simulink library "speedgoatlib_mscp"  (R2024b)
settings: Solver=VariableStepAuto  StartTime=0.0  StopTime=10.0  RelTol=1e-3
libraries: slrealtimeethercatlib x517, simulink x316, hdlsllib x168, $bdroot x11, slrealtimeutilitieslib x1
(part 3 of 5)

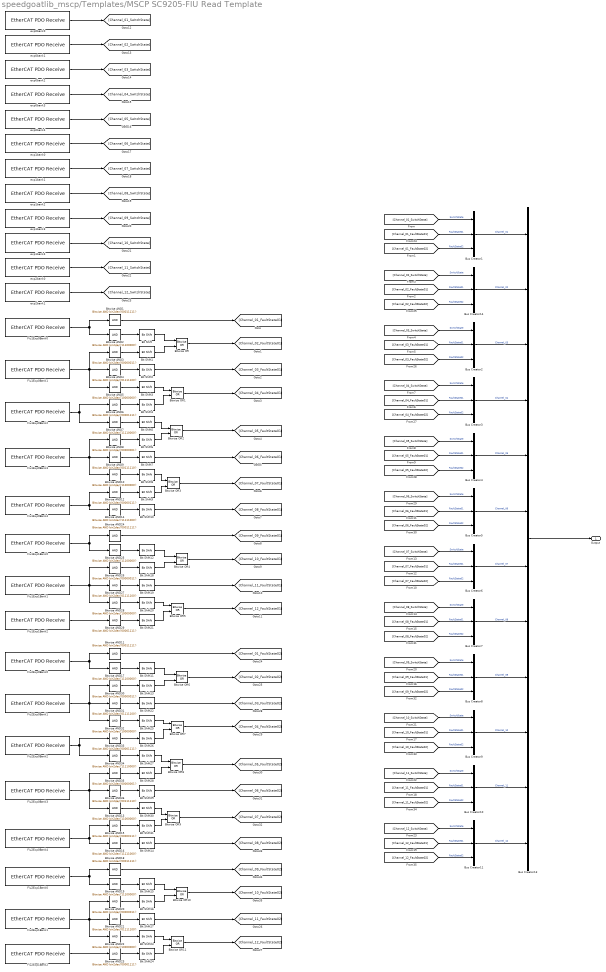
== system speedgoatlib_mscp/Templates/MSCP SC9205-FIU Read Template ==
  Bit Shift{,11..12,15} (4 alike) : hdlsllib/Logic and Bit Operations/Bit Shift  mode=Shift Right Logical  N=5
  Bit Shift{1,13,16,18} (4 alike) : hdlsllib/Logic and Bit Operations/Bit Shift  mode=Shift Left Logical  N=3
  Bit Shift10 : hdlsllib/Logic and Bit Operations/Bit Shift  mode=Shift Right Logical  N=3
  Bit Shift14 : hdlsllib/Logic and Bit Operations/Bit Shift  mode=Shift Right Logical  N=3
  Bit Shift{2,17,19,22} (4 alike) : hdlsllib/Logic and Bit Operations/Bit Shift  mode=Shift Right Logical  N=2
  Bit Shift{3,20,23,25} (4 alike) : hdlsllib/Logic and Bit Operations/Bit Shift  mode=Shift Right Logical  N=7
  Bit Shift{4,21,24,26} (4 alike) : hdlsllib/Logic and Bit Operations/Bit Shift  mode=Shift Left Logical  N=1
  Bit Shift27 : hdlsllib/Logic and Bit Operations/Bit Shift  mode=Shift Right Logical  N=4
  Bit Shift28 : hdlsllib/Logic and Bit Operations/Bit Shift  mode=Shift Left Logical  N=4
  Bit Shift29 : hdlsllib/Logic and Bit Operations/Bit Shift  mode=Shift Right Logical  N=1
  Bit Shift30 : hdlsllib/Logic and Bit Operations/Bit Shift  mode=Shift Right Logical  N=6
  Bit Shift31 : hdlsllib/Logic and Bit Operations/Bit Shift  mode=Shift Left Logical  N=2
  Bit Shift5 : hdlsllib/Logic and Bit Operations/Bit Shift  mode=Shift Right Logical  N=4
  Bit Shift6 : hdlsllib/Logic and Bit Operations/Bit Shift  mode=Shift Left Logical  N=4
  Bit Shift7 : hdlsllib/Logic and Bit Operations/Bit Shift  mode=Shift Right Logical  N=1
  Bit Shift8 : hdlsllib/Logic and Bit Operations/Bit Shift  mode=Shift Right Logical  N=6
  Bit Shift9 : hdlsllib/Logic and Bit Operations/Bit Shift  mode=Shift Left Logical  N=2
  Bitwise AND{1,11,18,24} (4 alike) : simulink/Logic and Bit Operations/Bitwise Operator  logicop=AND  UseBitMask=on  BitMask=bin2dec('00011111')  BitMaskRealWorld=Stored Integer
  Bitwise AND10 : simulink/Logic and Bit Operations/Bitwise Operator  logicop=AND  UseBitMask=on  BitMask=bin2dec('11000000')  BitMaskRealWorld=Stored Integer
  Bitwise AND12 : simulink/Logic and Bit Operations/Bitwise Operator  logicop=AND  UseBitMask=on  BitMask=bin2dec('00000111')  BitMaskRealWorld=Stored Integer
  Bitwise AND13 : simulink/Logic and Bit Operations/Bitwise Operator  logicop=AND  UseBitMask=on  BitMask=bin2dec('11000000')  BitMaskRealWorld=Stored Integer
  Bitwise AND14 : simulink/Logic and Bit Operations/Bitwise Operator  logicop=AND  UseBitMask=on  BitMask=bin2dec('11111000')  BitMaskRealWorld=Stored Integer
  Bitwise AND15 : simulink/Logic and Bit Operations/Bitwise Operator  logicop=AND  UseBitMask=on  BitMask=bin2dec('00000111')  BitMaskRealWorld=Stored Integer
  Bitwise AND16 : simulink/Logic and Bit Operations/Bitwise Operator  logicop=AND  UseBitMask=on  BitMask=bin2dec('11111000')  BitMaskRealWorld=Stored Integer
  Bitwise AND{2,17,19,25} (4 alike) : simulink/Logic and Bit Operations/Bitwise Operator  logicop=AND  UseBitMask=on  BitMask=bin2dec('11100000')  BitMaskRealWorld=Stored Integer
  Bitwise AND{3,20,26,30} (4 alike) : simulink/Logic and Bit Operations/Bitwise Operator  logicop=AND  UseBitMask=on  BitMask=bin2dec('00000011')  BitMaskRealWorld=Stored Integer
  Bitwise AND{4,21,27,31} (4 alike) : simulink/Logic and Bit Operations/Bitwise Operator  logicop=AND  UseBitMask=on  BitMask=bin2dec('01111100')  BitMaskRealWorld=Stored Integer
  Bitwise AND{5,22,28,32} (4 alike) : simulink/Logic and Bit Operations/Bitwise Operator  logicop=AND  UseBitMask=on  BitMask=bin2dec('10000000')  BitMaskRealWorld=Stored Integer
  Bitwise AND{6,23,29,33} (4 alike) : simulink/Logic and Bit Operations/Bitwise Operator  logicop=AND  UseBitMask=on  BitMask=bin2dec('00001111')  BitMaskRealWorld=Stored Integer
  Bitwise AND34 : simulink/Logic and Bit Operations/Bitwise Operator  logicop=AND  UseBitMask=on  BitMask=bin2dec('11110000')  BitMaskRealWorld=Stored Integer
  Bitwise AND35 : simulink/Logic and Bit Operations/Bitwise Operator  logicop=AND  UseBitMask=on  BitMask=bin2dec('00000001')  BitMaskRealWorld=Stored Integer
  Bitwise AND36 : simulink/Logic and Bit Operations/Bitwise Operator  logicop=AND  UseBitMask=on  BitMask=bin2dec('00111110')  BitMaskRealWorld=Stored Integer
  Bitwise AND7 : simulink/Logic and Bit Operations/Bitwise Operator  logicop=AND  UseBitMask=on  BitMask=bin2dec('11110000')  BitMaskRealWorld=Stored Integer
  Bitwise AND8 : simulink/Logic and Bit Operations/Bitwise Operator  logicop=AND  UseBitMask=on  BitMask=bin2dec('00000001')  BitMaskRealWorld=Stored Integer
  Bitwise AND9 : simulink/Logic and Bit Operations/Bitwise Operator  logicop=AND  UseBitMask=on  BitMask=bin2dec('00111110')  BitMaskRealWorld=Stored Integer
  Bitwise OR{,1..11} (12 alike) : simulink/Logic and Bit Operations/Bitwise Operator  logicop=OR  UseBitMask=off  NumInputPorts=2  BitMask=bin2dec('11011001')  BitMaskRealWorld=Stored Integer
  Bus Creator{1..11,14} (12 alike) : BusCreator  Inputs=3  OutDataTypeStr=Bus: MscpBus_SC9205_FIU_Channel
      settings: InheritFromInputs=off
  Bus Creator13 : BusCreator  Inputs=12  OutDataTypeStr=Bus: MscpBus_SC9205_FIU
      settings: InheritFromInputs=off
  Fiu1Exp0Bank{0..4} (5 alike) : slrealtimeethercatlib/EtherCAT PDO Receive  Priority=2  sig_name=Uninitialized Block  sig_offset=144  sig_type=uint8  type_size=8  sig_dim=1  device_id=0  sample_time=0.010000
  Fiu1Exp1Bank0 : slrealtimeethercatlib/EtherCAT PDO Receive  Priority=2  sig_name=Uninitialized Block  sig_offset=144  sig_type=uint8  type_size=8  sig_dim=1  device_id=0  sample_time=0.010000
  Fiu1Exp1Bank1 : slrealtimeethercatlib/EtherCAT PDO Receive  Priority=2  sig_name=Uninitialized Block  sig_offset=144  sig_type=uint8  type_size=8  sig_dim=1  device_id=0  sample_time=0.010000
  Fiu1Exp1Bank2 : slrealtimeethercatlib/EtherCAT PDO Receive  Priority=2  sig_name=Uninitialized Block  sig_offset=144  sig_type=uint8  type_size=8  sig_dim=1  device_id=0  sample_time=0.010000
  Fiu2Exp0Bank{0..4} (5 alike) : slrealtimeethercatlib/EtherCAT PDO Receive  Priority=2  sig_name=Uninitialized Block  sig_offset=144  sig_type=uint8  type_size=8  sig_dim=1  device_id=0  sample_time=0.010000
  Fiu2Exp1Bank0 : slrealtimeethercatlib/EtherCAT PDO Receive  Priority=2  sig_name=Uninitialized Block  sig_offset=144  sig_type=uint8  type_size=8  sig_dim=1  device_id=0  sample_time=0.010000
  Fiu2Exp1Bank1 : slrealtimeethercatlib/EtherCAT PDO Receive  Priority=2  sig_name=Uninitialized Block  sig_offset=144  sig_type=uint8  type_size=8  sig_dim=1  device_id=0  sample_time=0.010000
  Fiu2Exp1Bank2 : slrealtimeethercatlib/EtherCAT PDO Receive  Priority=2  sig_name=Uninitialized Block  sig_offset=144  sig_type=uint8  type_size=8  sig_dim=1  device_id=0  sample_time=0.010000
  exp0bank{0..4} (5 alike) : slrealtimeethercatlib/EtherCAT PDO Receive  Priority=2  sig_name=Uninitialized Block  sig_offset=144  sig_type=uint8  type_size=8  sig_dim=1  device_id=0  sample_time=0.010000
  exp1bank{0..4} (5 alike) : slrealtimeethercatlib/EtherCAT PDO Receive  Priority=2  sig_name=Uninitialized Block  sig_offset=144  sig_type=uint8  type_size=8  sig_dim=1  device_id=0  sample_time=0.010000
  exp2bank0 : slrealtimeethercatlib/EtherCAT PDO Receive  Priority=2  sig_name=Uninitialized Block  sig_offset=144  sig_type=uint8  type_size=8  sig_dim=1  device_id=0  sample_time=0.010000
  exp2bank1 : slrealtimeethercatlib/EtherCAT PDO Receive  Priority=2  sig_name=Uninitialized Block  sig_offset=144  sig_type=uint8  type_size=8  sig_dim=1  device_id=0  sample_time=0.010000
  Output : Outport
  wires:
  Bus Creator13/1 -> Output/1
  Fiu1Exp1Bank0/1 -> Bitwise AND25/1, Bitwise AND24/1
  Bitwise AND24/1 -> [Channel_09_FaultState01]
  Bit Shift18/1 -> Bitwise OR4/2
  Bit Shift12/1 -> Bitwise OR4/1
  Bitwise OR4/1 -> [Channel_10_FaultState01]
  Bitwise AND26/1 -> Bit Shift18/1
  Bitwise AND25/1 -> Bit Shift12/1
  Fiu1Exp1Bank1/1 -> Bitwise AND26/1, Bitwise AND28/1, Bitwise AND27/1
  Bitwise AND27/1 -> Bit Shift19/1
  Bit Shift19/1 -> [Channel_11_FaultState01]
  Bitwise AND28/1 -> Bit Shift20/1
  Bit Shift20/1 -> Bitwise OR5/1
  Fiu1Exp1Bank2/1 -> Bitwise AND29/1
  Bitwise AND29/1 -> Bit Shift21/1
  Bit Shift21/1 -> Bitwise OR5/2
  Bitwise OR5/1 -> [Channel_12_FaultState01]
  Bit Shift10/1 -> [Channel_08_FaultState01]
  Bitwise AND14/1 -> Bit Shift10/1
  Bitwise OR3/1 -> [Channel_07_FaultState01]
  Bit Shift9/1 -> Bitwise OR3/2
  Bit Shift8/1 -> Bitwise OR3/1
  Bitwise AND12/1 -> Bit Shift9/1
  Fiu1Exp0Bank4/1 -> Bitwise AND12/1, Bitwise AND14/1
  Bitwise AND10/1 -> Bit Shift8/1
  Bit Shift7/1 -> [Channel_06_FaultState01]
  Bitwise AND9/1 -> Bit Shift7/1
  Bitwise OR2/1 -> [Channel_05_FaultState01]
  Fiu1Exp0Bank3/1 -> Bitwise AND8/1, Bitwise AND9/1, Bitwise AND10/1
  Bitwise AND8/1 -> Bit Shift6/1
  Bit Shift6/1 -> Bitwise OR2/2
  Bit Shift5/1 -> Bitwise OR2/1
  Bitwise AND7/1 -> Bit Shift5/1
  Bitwise OR1/1 -> [Channel_04_FaultState01]
  Bit Shift4/1 -> Bitwise OR1/2
  Bitwise AND6/1 -> Bit Shift4/1
  Fiu1Exp0Bank2/1 -> Bitwise AND7/1, Bitwise AND6/1
  Bit Shift3/1 -> Bitwise OR1/1
  Bitwise AND5/1 -> Bit Shift3/1
  Bit Shift2/1 -> [Channel_03_FaultState01]
  Bitwise AND4/1 -> Bit Shift2/1
  Fiu1Exp0Bank1/1 -> Bitwise AND4/1, Bitwise AND5/1, Bitwise AND3/1
  Bitwise AND2/1 -> Bit Shift/1
  Bitwise AND3/1 -> Bit Shift1/1
  Bitwise OR/1 -> [Channel_02_FaultState01]
  Bit Shift/1 -> Bitwise OR/1
  Bit Shift1/1 -> Bitwise OR/2
  Bitwise AND1/1 -> [Channel_01_FaultState01]
  Fiu1Exp0Bank0/1 -> Bitwise AND1/1, Bitwise AND2/1
  exp0bank0/1 -> [Channel_01_SwitchState]
  exp0bank1/1 -> [Channel_02_SwitchState]
  exp0bank2/1 -> [Channel_03_SwitchState]
  exp0bank3/1 -> [Channel_04_SwitchState]
  exp0bank4/1 -> [Channel_05_SwitchState]
  exp1bank0/1 -> [Channel_06_SwitchState]
  exp1bank1/1 -> [Channel_07_SwitchState]
  exp1bank2/1 -> [Channel_08_SwitchState]
  exp1bank3/1 -> [Channel_09_SwitchState]
  exp1bank4/1 -> [Channel_10_SwitchState]
  exp2bank0/1 -> [Channel_11_SwitchState]
  exp2bank1/1 -> [Channel_12_SwitchState]
  Fiu2Exp0Bank0/1 -> Bitwise AND17/1, Bitwise AND11/1
  Bitwise AND11/1 -> [Channel_01_FaultState02]
  Bit Shift13/1 -> Bitwise OR6/2
  Bit Shift11/1 -> Bitwise OR6/1
  Bitwise OR6/1 -> [Channel_02_FaultState02]
  Bitwise AND30/1 -> Bit Shift13/1
  Bitwise AND17/1 -> Bit Shift11/1
  Fiu2Exp0Bank1/1 -> Bitwise AND30/1, Bitwise AND32/1, Bitwise AND31/1
  Bitwise AND31/1 -> Bit Shift22/1
  Bit Shift22/1 -> [Channel_03_FaultState02]
  Bitwise AND32/1 -> Bit Shift25/1
  Bit Shift25/1 -> Bitwise OR7/1
  Fiu2Exp0Bank2/1 -> Bitwise AND33/1, Bitwise AND34/1
  Bitwise AND33/1 -> Bit Shift26/1
  Bit Shift26/1 -> Bitwise OR7/2
  Bitwise OR7/1 -> [Channel_04_FaultState02]
  Bitwise AND34/1 -> Bit Shift27/1
  Bit Shift27/1 -> Bitwise OR8/1
  Bit Shift28/1 -> Bitwise OR8/2
  Bitwise AND35/1 -> Bit Shift28/1
  Fiu2Exp0Bank3/1 -> Bitwise AND13/1, Bitwise AND36/1, Bitwise AND35/1
  Bitwise OR8/1 -> [Channel_05_FaultState02]
  Bitwise AND36/1 -> Bit Shift29/1
  Bit Shift29/1 -> [Channel_06_FaultState02]
  Bitwise AND13/1 -> Bit Shift30/1
  Fiu2Exp0Bank4/1 -> Bitwise AND16/1, Bitwise AND15/1
  Bitwise AND15/1 -> Bit Shift31/1
  Bit Shift30/1 -> Bitwise OR9/1
  Bit Shift31/1 -> Bitwise OR9/2
  Bitwise OR9/1 -> [Channel_07_FaultState02]
  Bitwise AND16/1 -> Bit Shift14/1
  Bit Shift14/1 -> [Channel_08_FaultState02]
  Bitwise OR11/1 -> [Channel_12_FaultState02]
  Bit Shift24/1 -> Bitwise OR11/2
  Bitwise AND23/1 -> Bit Shift24/1
  Fiu2Exp1Bank2/1 -> Bitwise AND23/1
  Bit Shift23/1 -> Bitwise OR11/1
  Bitwise AND22/1 -> Bit Shift23/1
  Bit Shift17/1 -> [Channel_11_FaultState02]
  Bitwise AND21/1 -> Bit Shift17/1
  Fiu2Exp1Bank1/1 -> Bitwise AND21/1, Bitwise AND22/1, Bitwise AND20/1
  Bitwise AND19/1 -> Bit Shift15/1
  Bitwise AND20/1 -> Bit Shift16/1
  Bitwise OR10/1 -> [Channel_10_FaultState02]
  Bit Shift15/1 -> Bitwise OR10/1
  Bit Shift16/1 -> Bitwise OR10/2
  Bitwise AND18/1 -> [Channel_09_FaultState02]
  Fiu2Exp1Bank0/1 -> Bitwise AND18/1, Bitwise AND19/1
  Bus Creator1/1 -> Bus Creator13/1  "Channel_01"
  [Channel_01_SwitchState] -> Bus Creator1/1  "SwitchState"
  [Channel_01_FaultState01] -> Bus Creator1/2  "FaultState01"
  [Channel_01_FaultState02] -> Bus Creator1/3  "FaultState02"
  Bus Creator14/1 -> Bus Creator13/2  "Channel_02"
  [Channel_02_SwitchState] -> Bus Creator14/1  "SwitchState"
  [Channel_02_FaultState01] -> Bus Creator14/2  "FaultState01"
  [Channel_02_FaultState02] -> Bus Creator14/3  "FaultState02"
  Bus Creator2/1 -> Bus Creator13/3  "Channel_03"
  [Channel_03_FaultState02] -> Bus Creator2/3  "FaultState02"
  [Channel_03_FaultState01] -> Bus Creator2/2  "FaultState01"
  [Channel_03_SwitchState] -> Bus Creator2/1  "SwitchState"
  Bus Creator3/1 -> Bus Creator13/4  "Channel_04"
  [Channel_04_SwitchState] -> Bus Creator3/1  "SwitchState"
  [Channel_04_FaultState02] -> Bus Creator3/3  "FaultState02"
  [Channel_04_FaultState01] -> Bus Creator3/2  "FaultState01"
  Bus Creator4/1 -> Bus Creator13/5  "Channel_05"
  [Channel_05_SwitchState] -> Bus Creator4/1  "SwitchState"
  [Channel_05_FaultState01] -> Bus Creator4/2  "FaultState01"
  [Channel_05_FaultState02] -> Bus Creator4/3  "FaultState02"
  Bus Creator5/1 -> Bus Creator13/6  "Channel_06"
  [Channel_06_SwitchState] -> Bus Creator5/1  "SwitchState"
  [Channel_06_FaultState01] -> Bus Creator5/2  "FaultState01"
  [Channel_06_FaultState02] -> Bus Creator5/3  "FaultState02"
  Bus Creator6/1 -> Bus Creator13/7  "Channel_07"
  [Channel_07_FaultState01] -> Bus Creator6/2  "FaultState01"
  [Channel_07_FaultState02] -> Bus Creator6/3  "FaultState02"
  [Channel_07_SwitchState] -> Bus Creator6/1  "SwitchState"
  Bus Creator7/1 -> Bus Creator13/8  "Channel_08"
  [Channel_08_SwitchState] -> Bus Creator7/1  "SwitchState"
  [Channel_08_FaultState01] -> Bus Creator7/2  "FaultState01"
  [Channel_08_FaultState02] -> Bus Creator7/3  "FaultState02"
  Bus Creator8/1 -> Bus Creator13/9  "Channel_09"
  [Channel_09_SwitchState] -> Bus Creator8/1  "SwitchState"
  [Channel_09_FaultState01] -> Bus Creator8/2  "FaultState01"
  [Channel_09_FaultState02] -> Bus Creator8/3  "FaultState02"
  Bus Creator9/1 -> Bus Creator13/10  "Channel_10"
  [Channel_10_SwitchState] -> Bus Creator9/1  "SwitchState"
  [Channel_10_FaultState01] -> Bus Creator9/2  "FaultState01"
  [Channel_10_FaultState02] -> Bus Creator9/3  "FaultState02"
  Bus Creator10/1 -> Bus Creator13/11  "Channel_11"
  [Channel_11_SwitchState] -> Bus Creator10/1  "SwitchState"
  [Channel_11_FaultState01] -> Bus Creator10/2  "FaultState01"
  [Channel_11_FaultState02] -> Bus Creator10/3  "FaultState02"
  Bus Creator11/1 -> Bus Creator13/12  "Channel_12"
  [Channel_12_SwitchState] -> Bus Creator11/1  "SwitchState"
  [Channel_12_FaultState01] -> Bus Creator11/2  "FaultState01"
  [Channel_12_FaultState02] -> Bus Creator11/3  "FaultState02"

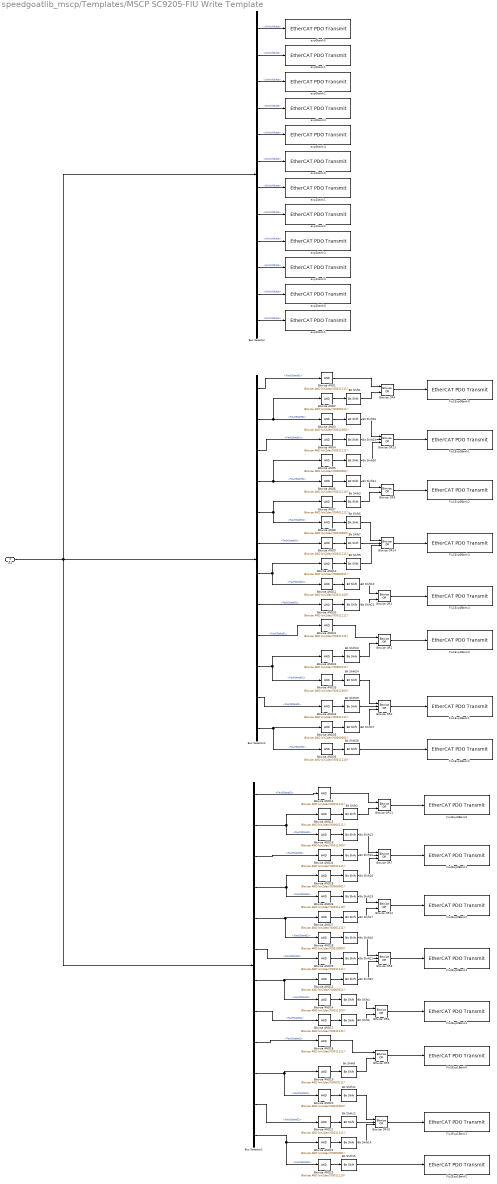
== system speedgoatlib_mscp/Templates/MSCP SC9205-FIU Write Template ==
  In1 : Inport  OutDataTypeStr=Bus: MscpBus_SC9205_FIU
  Bit Shift{1..2,8,23} (4 alike) : hdlsllib/Logic and Bit Operations/Bit Shift  mode=Shift Left Logical  N=5
  Bit Shift10 : hdlsllib/Logic and Bit Operations/Bit Shift  mode=Shift Right Logical  N=2
  Bit Shift{11,13,24,26} (4 alike) : hdlsllib/Logic and Bit Operations/Bit Shift  mode=Shift Right Logical  N=3
  Bit Shift{12,16,25,29} (4 alike) : hdlsllib/Logic and Bit Operations/Bit Shift  mode=Shift Left Logical  N=2
  Bit Shift{14,18,27,30} (4 alike) : hdlsllib/Logic and Bit Operations/Bit Shift  mode=Shift Left Logical  N=7
  Bit Shift{15,19,28,31} (4 alike) : hdlsllib/Logic and Bit Operations/Bit Shift  mode=Shift Right Logical  N=1
  Bit Shift17 : hdlsllib/Logic and Bit Operations/Bit Shift  mode=Shift Left Logical  N=4
  Bit Shift20 : hdlsllib/Logic and Bit Operations/Bit Shift  mode=Shift Right Logical  N=4
  Bit Shift21 : hdlsllib/Logic and Bit Operations/Bit Shift  mode=Shift Left Logical  N=1
  Bit Shift22 : hdlsllib/Logic and Bit Operations/Bit Shift  mode=Shift Left Logical  N=3
  Bit Shift3 : hdlsllib/Logic and Bit Operations/Bit Shift  mode=Shift Left Logical  N=4
  Bit Shift32 : hdlsllib/Logic and Bit Operations/Bit Shift  mode=Shift Left Logical  N=6
  Bit Shift4 : hdlsllib/Logic and Bit Operations/Bit Shift  mode=Shift Right Logical  N=2
  Bit Shift5 : hdlsllib/Logic and Bit Operations/Bit Shift  mode=Shift Right Logical  N=4
  Bit Shift6 : hdlsllib/Logic and Bit Operations/Bit Shift  mode=Shift Left Logical  N=3
  Bit Shift7 : hdlsllib/Logic and Bit Operations/Bit Shift  mode=Shift Left Logical  N=1
  Bit Shift9 : hdlsllib/Logic and Bit Operations/Bit Shift  mode=Shift Left Logical  N=6
  Bitwise AND{1,4,9,12,17..18,21,24,29..31,34} (12 alike) : simulink/Logic and Bit Operations/Bitwise Operator  logicop=AND  UseBitMask=on  BitMask=bin2dec('00011111')  BitMaskRealWorld=Stored Integer
      settings: LibrarySourceBlock=|
      | simulink/Quick Insert/Logic and Bit
      | Operations/Bitwise AND
  Bitwise AND10 : simulink/Logic and Bit Operations/Bitwise Operator  logicop=AND  UseBitMask=on  BitMask=bin2dec('00000011')  BitMaskRealWorld=Stored Integer
      settings: LibrarySourceBlock=|
      | simulink/Quick Insert/Logic and Bit
      | Operations/Bitwise AND
  Bitwise AND11 : simulink/Logic and Bit Operations/Bitwise Operator  logicop=AND  UseBitMask=on  BitMask=bin2dec('00011100')  BitMaskRealWorld=Stored Integer
      settings: LibrarySourceBlock=|
      | simulink/Quick Insert/Logic and Bit
      | Operations/Bitwise AND
  Bitwise AND13 : simulink/Logic and Bit Operations/Bitwise Operator  logicop=AND  UseBitMask=on  BitMask=bin2dec('00000011')  BitMaskRealWorld=Stored Integer
      settings: LibrarySourceBlock=|
      | simulink/Quick Insert/Logic and Bit
      | Operations/Bitwise AND
  Bitwise AND14 : simulink/Logic and Bit Operations/Bitwise Operator  logicop=AND  UseBitMask=on  BitMask=bin2dec('00011100')  BitMaskRealWorld=Stored Integer
      settings: LibrarySourceBlock=|
      | simulink/Quick Insert/Logic and Bit
      | Operations/Bitwise AND
  Bitwise AND{2,15,19,32} (4 alike) : simulink/Logic and Bit Operations/Bitwise Operator  logicop=AND  UseBitMask=on  BitMask=bin2dec('00000111')  BitMaskRealWorld=Stored Integer
      settings: LibrarySourceBlock=|
      | simulink/Quick Insert/Logic and Bit
      | Operations/Bitwise AND
  Bitwise AND{3,16,20,33} (4 alike) : simulink/Logic and Bit Operations/Bitwise Operator  logicop=AND  UseBitMask=on  BitMask=bin2dec('00011000')  BitMaskRealWorld=Stored Integer
      settings: LibrarySourceBlock=|
      | simulink/Quick Insert/Logic and Bit
      | Operations/Bitwise AND
  Bitwise AND{5,22,25,35} (4 alike) : simulink/Logic and Bit Operations/Bitwise Operator  logicop=AND  UseBitMask=on  BitMask=bin2dec('00000001')  BitMaskRealWorld=Stored Integer
      settings: LibrarySourceBlock=|
      | simulink/Quick Insert/Logic and Bit
      | Operations/Bitwise AND
  Bitwise AND{6,23,26,36} (4 alike) : simulink/Logic and Bit Operations/Bitwise Operator  logicop=AND  UseBitMask=on  BitMask=bin2dec('00011110')  BitMaskRealWorld=Stored Integer
      settings: LibrarySourceBlock=|
      | simulink/Quick Insert/Logic and Bit
      | Operations/Bitwise AND
  Bitwise AND27 : simulink/Logic and Bit Operations/Bitwise Operator  logicop=AND  UseBitMask=on  BitMask=bin2dec('00001111')  BitMaskRealWorld=Stored Integer
      settings: LibrarySourceBlock=|
      | simulink/Quick Insert/Logic and Bit
      | Operations/Bitwise AND
  Bitwise AND28 : simulink/Logic and Bit Operations/Bitwise Operator  logicop=AND  UseBitMask=on  BitMask=bin2dec('00010000')  BitMaskRealWorld=Stored Integer
      settings: LibrarySourceBlock=|
      | simulink/Quick Insert/Logic and Bit
      | Operations/Bitwise AND
  Bitwise AND7 : simulink/Logic and Bit Operations/Bitwise Operator  logicop=AND  UseBitMask=on  BitMask=bin2dec('00001111')  BitMaskRealWorld=Stored Integer
      settings: LibrarySourceBlock=|
      | simulink/Quick Insert/Logic and Bit
      | Operations/Bitwise AND
  Bitwise AND8 : simulink/Logic and Bit Operations/Bitwise Operator  logicop=AND  UseBitMask=on  BitMask=bin2dec('00010000')  BitMaskRealWorld=Stored Integer
      settings: LibrarySourceBlock=|
      | simulink/Quick Insert/Logic and Bit
      | Operations/Bitwise AND
  Bitwise OR{1..2,4..6,9,11..12} (8 alike) : simulink/Logic and Bit Operations/Bitwise Operator  logicop=OR  UseBitMask=off  NumInputPorts=2  BitMask=bin2dec('11011001')  BitMaskRealWorld=Stored Integer
      settings: LibrarySourceBlock=|
      | simulink/Quick Insert/Logic and Bit
      | Operations/Bitwise OR
  Bitwise OR{3,7..8,10,13..14} (6 alike) : simulink/Logic and Bit Operations/Bitwise Operator  logicop=OR  UseBitMask=off  NumInputPorts=3  BitMask=bin2dec('11011001')  BitMaskRealWorld=Stored Integer
      settings: LibrarySourceBlock=|
      | simulink/Quick Insert/Logic and Bit
      | Operations/Bitwise OR
  Bus Selector : BusSelector  OutputSignals=Channel_01.SwitchState,Channel_02.SwitchState,Channel_03.SwitchState,Channel_04.SwitchState,Channel_05.SwitchState,Channel_06.SwitchState,Channel_07.SwitchState,Channel_08.SwitchState,Channel_09.SwitchState,Channel_10.SwitchState,Channel_11.SwitchState,Channel_12.SwitchState
  Bus Selector1 : BusSelector  OutputSignals=Channel_01.FaultState02,Channel_02.FaultState02,Channel_03.FaultState02,Channel_04.FaultState02,Channel_05.FaultState02,Channel_06.FaultState02,Channel_07.FaultState02,Channel_08.FaultState02,Channel_09.FaultState02,Channel_10.FaultState02,Channel_11.FaultState02,Channel_12.FaultState02
  Bus Selector2 : BusSelector  OutputSignals=Channel_01.FaultState01,Channel_02.FaultState01,Channel_03.FaultState01,Channel_04.FaultState01,Channel_05.FaultState01,Channel_06.FaultState01,Channel_07.FaultState01,Channel_08.FaultState01,Channel_09.FaultState01,Channel_10.FaultState01,Channel_11.FaultState01,Channel_12.FaultState01
  Fiu1Exp0Bank{0..4} (5 alike) : slrealtimeethercatlib/EtherCAT PDO Transmit  Priority=3  sig_name=Uninitialized Block  sig_offset=128  sig_type=uint8  type_size=8  sig_dim=1  device_id=0  sample_time=0.010000
  Fiu1Exp1Bank0 : slrealtimeethercatlib/EtherCAT PDO Transmit  Priority=3  sig_name=Uninitialized Block  sig_offset=128  sig_type=uint8  type_size=8  sig_dim=1  device_id=0  sample_time=0.010000
  Fiu1Exp1Bank1 : slrealtimeethercatlib/EtherCAT PDO Transmit  Priority=3  sig_name=Uninitialized Block  sig_offset=128  sig_type=uint8  type_size=8  sig_dim=1  device_id=0  sample_time=0.010000
  Fiu1Exp1Bank2 : slrealtimeethercatlib/EtherCAT PDO Transmit  Priority=3  sig_name=Uninitialized Block  sig_offset=128  sig_type=uint8  type_size=8  sig_dim=1  device_id=0  sample_time=0.010000
  Fiu2Exp0Bank{0..4} (5 alike) : slrealtimeethercatlib/EtherCAT PDO Transmit  Priority=3  sig_name=Uninitialized Block  sig_offset=128  sig_type=uint8  type_size=8  sig_dim=1  device_id=0  sample_time=0.010000
  Fiu2Exp1Bank0 : slrealtimeethercatlib/EtherCAT PDO Transmit  Priority=3  sig_name=Uninitialized Block  sig_offset=128  sig_type=uint8  type_size=8  sig_dim=1  device_id=0  sample_time=0.010000
  Fiu2Exp1Bank1 : slrealtimeethercatlib/EtherCAT PDO Transmit  Priority=3  sig_name=Uninitialized Block  sig_offset=128  sig_type=uint8  type_size=8  sig_dim=1  device_id=0  sample_time=0.010000
  Fiu2Exp1Bank2 : slrealtimeethercatlib/EtherCAT PDO Transmit  Priority=3  sig_name=Uninitialized Block  sig_offset=128  sig_type=uint8  type_size=8  sig_dim=1  device_id=0  sample_time=0.010000
  exp0bank{0..4} (5 alike) : slrealtimeethercatlib/EtherCAT PDO Transmit  Priority=3  sig_name=Uninitialized Block  sig_offset=128  sig_type=uint8  type_size=8  sig_dim=1  device_id=0  sample_time=0.010000
  exp1bank{0..4} (5 alike) : slrealtimeethercatlib/EtherCAT PDO Transmit  Priority=3  sig_name=Uninitialized Block  sig_offset=128  sig_type=uint8  type_size=8  sig_dim=1  device_id=0  sample_time=0.010000
  exp2bank0 : slrealtimeethercatlib/EtherCAT PDO Transmit  Priority=3  sig_name=Uninitialized Block  sig_offset=128  sig_type=uint8  type_size=8  sig_dim=1  device_id=0  sample_time=0.010000
  exp2bank1 : slrealtimeethercatlib/EtherCAT PDO Transmit  Priority=3  sig_name=Uninitialized Block  sig_offset=128  sig_type=uint8  type_size=8  sig_dim=1  device_id=0  sample_time=0.010000
  wires:
  Bus Selector/6 -> exp1bank0/1  "<SwitchState>"
  Bus Selector/5 -> exp0bank4/1  "<SwitchState>"
  Bus Selector/7 -> exp1bank1/1  "<SwitchState>"
  Bus Selector/8 -> exp1bank2/1  "<SwitchState>"
  Bus Selector/2 -> exp0bank1/1  "<SwitchState>"
  Bus Selector/4 -> exp0bank3/1  "<SwitchState>"
  Bus Selector/12 -> exp2bank1/1  "<SwitchState>"
  Bus Selector/9 -> exp1bank3/1  "<SwitchState>"
  Bus Selector/1 -> exp0bank0/1  "<SwitchState>"
  Bus Selector/11 -> exp2bank0/1  "<SwitchState>"
  Bus Selector/10 -> exp1bank4/1  "<SwitchState>"
  Bus Selector/3 -> exp0bank2/1  "<SwitchState>"
  Bitwise OR4/1 -> Fiu1Exp0Bank0/1
  Bitwise AND1/1 -> Bitwise OR4/1
  Bitwise OR3/1 -> Fiu1Exp1Bank1/1
  Bitwise AND10/1 -> Bit Shift9/1
  Bit Shift7/1 -> Bitwise OR14/2
  Bit Shift27/1 -> Bitwise OR3/3
  Bitwise AND31/1 -> Bitwise OR2/1
  Bus Selector2/12 -> Bitwise AND35/1, Bitwise AND36/1  "<FaultState01>"
  Bit Shift30/1 -> Bitwise OR13/3
  Bit Shift1/1 -> Bitwise OR4/2
  Bus Selector2/2 -> Bitwise AND2/1, Bitwise AND3/1  "<FaultState01>"
  Bit Shift28/1 -> Fiu1Exp1Bank2/1
  Bitwise AND36/1 -> Bit Shift28/1
  Bit Shift22/1 -> Bitwise OR1/2
  Bitwise AND11/1 -> Bit Shift10/1
  Bit Shift31/1 -> Bitwise OR5/1
  Bitwise AND4/1 -> Bit Shift29/1
  Bitwise AND30/1 -> Bit Shift22/1
  Bit Shift23/1 -> Bitwise OR2/2
  Bitwise OR5/1 -> Fiu1Exp0Bank2/1
  Bitwise OR2/1 -> Fiu1Exp1Bank0/1
  Bus Selector2/8 -> Bitwise AND30/1  "<FaultState01>"
  Bitwise AND33/1 -> Bit Shift24/1
  Bus Selector2/9 -> Bitwise AND31/1  "<FaultState01>"
  Bitwise AND3/1 -> Bit Shift26/1
  Bus Selector2/5 -> Bitwise AND7/1, Bitwise AND8/1  "<FaultState01>"
  Bit Shift24/1 -> Bitwise OR3/1
  Bit Shift29/1 -> Bitwise OR13/2
  Bitwise AND35/1 -> Bit Shift27/1
  Bus Selector2/3 -> Bitwise AND4/1  "<FaultState01>"
  Bit Shift10/1 -> Bitwise OR1/1
  Bit Shift5/1 -> Bitwise OR14/1
  Bus Selector2/1 -> Bitwise AND1/1  "<FaultState01>"
  Bus Selector2/7 -> Bitwise AND10/1, Bitwise AND11/1  "<FaultState01>"
  Bitwise OR14/1 -> Fiu1Exp0Bank3/1
  Bit Shift26/1 -> Bitwise OR13/1
  Bitwise OR13/1 -> Fiu1Exp0Bank1/1
  Bus Selector2/4 -> Bitwise AND5/1, Bitwise AND6/1  "<FaultState01>"
  Bitwise AND6/1 -> Bit Shift31/1
  Bit Shift25/1 -> Bitwise OR3/2
  Bit Shift3/1 -> Bitwise OR5/2
  Bitwise AND34/1 -> Bit Shift25/1
  Bit Shift9/1 -> Bitwise OR14/3
  Bitwise AND2/1 -> Bit Shift1/1
  Bitwise AND8/1 -> Bit Shift5/1
  Bitwise AND7/1 -> Bit Shift3/1
  Bitwise OR1/1 -> Fiu1Exp0Bank4/1
  Bitwise AND5/1 -> Bit Shift30/1
  Bus Selector2/10 -> Bitwise AND32/1, Bitwise AND33/1  "<FaultState01>"
  Bitwise AND32/1 -> Bit Shift23/1
  Bus Selector2/11 -> Bitwise AND34/1  "<FaultState01>"
  Bus Selector2/6 -> Bitwise AND9/1  "<FaultState01>"
  Bitwise AND9/1 -> Bit Shift7/1
  In1/1 -> Bus Selector/1, Bus Selector1/1, Bus Selector2/1
  Bitwise AND27/1 -> Bit Shift17/1
  Bitwise AND15/1 -> Bit Shift2/1
  Bitwise AND25/1 -> Bit Shift18/1
  Bitwise AND19/1 -> Bit Shift8/1
  Bus Selector1/11 -> Bitwise AND21/1  "<FaultState02>"
  Bitwise OR6/1 -> Fiu2Exp0Bank4/1
  Bus Selector1/6 -> Bitwise AND29/1  "<FaultState02>"
  Bitwise AND26/1 -> Bit Shift19/1
  Bus Selector1/4 -> Bitwise AND25/1, Bitwise AND26/1  "<FaultState02>"
  Bitwise AND21/1 -> Bit Shift12/1
  Bit Shift32/1 -> Bitwise OR8/3
  Bit Shift12/1 -> Bitwise OR10/2
  Bus Selector1/10 -> Bitwise AND19/1, Bitwise AND20/1  "<FaultState02>"
  Bit Shift13/1 -> Bitwise OR7/1
  Bit Shift11/1 -> Bitwise OR10/1
  Bus Selector1/3 -> Bitwise AND24/1  "<FaultState02>"
  Bus Selector1/1 -> Bitwise AND12/1  "<FaultState02>"
  Bitwise AND22/1 -> Bit Shift14/1
  Bit Shift20/1 -> Bitwise OR8/1
  Bit Shift4/1 -> Bitwise OR6/1
  Bus Selector1/5 -> Bitwise AND27/1, Bitwise AND28/1  "<FaultState02>"
  Bit Shift16/1 -> Bitwise OR7/2
  Bitwise AND16/1 -> Bit Shift13/1
  Bitwise OR8/1 -> Fiu2Exp0Bank3/1
  Bus Selector1/8 -> Bitwise AND17/1  "<FaultState02>"
  Bus Selector1/9 -> Bitwise AND18/1  "<FaultState02>"
  Bitwise OR7/1 -> Fiu2Exp0Bank1/1
  Bitwise OR9/1 -> Fiu2Exp1Bank0/1
  Bitwise OR12/1 -> Fiu2Exp0Bank2/1
  Bitwise AND28/1 -> Bit Shift20/1
  Bit Shift8/1 -> Bitwise OR9/2
  Bitwise AND24/1 -> Bit Shift16/1
  Bit Shift17/1 -> Bitwise OR12/2
  Bitwise AND14/1 -> Bit Shift4/1
  Bus Selector1/2 -> Bitwise AND15/1, Bitwise AND16/1  "<FaultState02>"
  Bit Shift2/1 -> Bitwise OR11/2
  Bit Shift6/1 -> Bitwise OR6/2
  Bit Shift15/1 -> Fiu2Exp1Bank2/1
  Bit Shift18/1 -> Bitwise OR7/3
  Bitwise AND23/1 -> Bit Shift15/1
  Bitwise AND20/1 -> Bit Shift11/1
  Bus Selector1/7 -> Bitwise AND13/1, Bitwise AND14/1  "<FaultState02>"
  Bus Selector1/12 -> Bitwise AND22/1, Bitwise AND23/1  "<FaultState02>"
  Bitwise AND13/1 -> Bit Shift32/1
  Bitwise AND12/1 -> Bitwise OR11/1
  Bitwise AND17/1 -> Bit Shift6/1
  Bit Shift19/1 -> Bitwise OR12/1
  Bitwise OR10/1 -> Fiu2Exp1Bank1/1
  Bit Shift21/1 -> Bitwise OR8/2
  Bitwise AND18/1 -> Bitwise OR9/1
  Bitwise OR11/1 -> Fiu2Exp0Bank0/1
  Bitwise AND29/1 -> Bit Shift21/1
  Bit Shift14/1 -> Bitwise OR10/3

== system speedgoatlib_mscp/Templates/MSCP SC9502-SPDT-TTL Read Template ==
  Bus Creator : BusCreator  Inputs=16  OutDataTypeStr=Bus: MscpBus_SC9502_SPDT_TTL
      settings: InheritFromInputs=off
  S-Function1 : S-Function  FunctionName=sg_mscp_SC9502_SPDT_TTL_read  SFunctionDeploymentMode=off  EnableBusSupport=off
  exp0bank0 : slrealtimeethercatlib/EtherCAT PDO Receive  Priority=2  sig_name=Uninitialized Block  sig_offset=144  sig_type=uint8  type_size=8  sig_dim=1  device_id=0  sample_time=0.010000
  exp0bank1 : slrealtimeethercatlib/EtherCAT PDO Receive  Priority=2  sig_name=Uninitialized Block  sig_offset=144  sig_type=uint8  type_size=8  sig_dim=1  device_id=0  sample_time=0.010000
  Out1 : Outport
  wires:
  exp0bank0/1 -> S-Function1/1
  exp0bank1/1 -> S-Function1/2
  Bus Creator/1 -> Out1/1
  S-Function1/1 -> Bus Creator/1  "Channel_01"
  S-Function1/2 -> Bus Creator/2  "Channel_02"
  S-Function1/3 -> Bus Creator/3  "Channel_03"
  S-Function1/4 -> Bus Creator/4  "Channel_04"
  S-Function1/5 -> Bus Creator/5  "Channel_05"
  S-Function1/6 -> Bus Creator/6  "Channel_06"
  S-Function1/7 -> Bus Creator/7  "Channel_07"
  S-Function1/8 -> Bus Creator/8  "Channel_08"
  S-Function1/9 -> Bus Creator/9  "Channel_09"
  S-Function1/10 -> Bus Creator/10  "Channel_10"
  S-Function1/11 -> Bus Creator/11  "Channel_11"
  S-Function1/12 -> Bus Creator/12  "Channel_12"
  S-Function1/13 -> Bus Creator/13  "Channel_13"
  S-Function1/14 -> Bus Creator/14  "Channel_14"
  S-Function1/15 -> Bus Creator/15  "Channel_15"
  S-Function1/16 -> Bus Creator/16  "Channel_16"

== system speedgoatlib_mscp/Templates/MSCP SC9502-SPDT-TTL Write Template ==
  In2 : Inport  OutDataTypeStr=Bus: MscpBus_SC9502_SPDT_TTL
  Bus Selector1 : BusSelector  OutputSignals=Channel_01,Channel_02,Channel_03,Channel_04,Channel_05,Channel_06,Channel_07,Channel_08,Channel_09,Channel_10,Channel_11,Channel_12,Channel_13,Channel_14,Channel_15,Channel_16
  S-Function1 : S-Function  FunctionName=sg_mscp_SC9502_SPDT_TTL_write  SFunctionDeploymentMode=off  EnableBusSupport=off
  exp0bank0 : slrealtimeethercatlib/EtherCAT PDO Transmit  Priority=3  sig_name=Uninitialized Block  sig_offset=128  sig_type=uint8  type_size=8  sig_dim=1  device_id=0  sample_time=0.010000
  exp0bank1 : slrealtimeethercatlib/EtherCAT PDO Transmit  Priority=3  sig_name=Uninitialized Block  sig_offset=128  sig_type=uint8  type_size=8  sig_dim=1  device_id=0  sample_time=0.010000
  wires:
  Bus Selector1/1 -> S-Function1/1  "<Channel_01>"
  In2/1 -> Bus Selector1/1
  Bus Selector1/2 -> S-Function1/2  "<Channel_02>"
  Bus Selector1/3 -> S-Function1/3  "<Channel_03>"
  Bus Selector1/4 -> S-Function1/4  "<Channel_04>"
  Bus Selector1/5 -> S-Function1/5  "<Channel_05>"
  Bus Selector1/6 -> S-Function1/6  "<Channel_06>"
  Bus Selector1/7 -> S-Function1/7  "<Channel_07>"
  Bus Selector1/8 -> S-Function1/8  "<Channel_08>"
  Bus Selector1/9 -> S-Function1/9  "<Channel_09>"
  Bus Selector1/10 -> S-Function1/10  "<Channel_10>"
  Bus Selector1/11 -> S-Function1/11  "<Channel_11>"
  Bus Selector1/12 -> S-Function1/12  "<Channel_12>"
  Bus Selector1/13 -> S-Function1/13  "<Channel_13>"
  Bus Selector1/14 -> S-Function1/14  "<Channel_14>"
  Bus Selector1/15 -> S-Function1/15  "<Channel_15>"
  Bus Selector1/16 -> S-Function1/16  "<Channel_16>"
  S-Function1/1 -> exp0bank0/1
  S-Function1/2 -> exp0bank1/1

== system speedgoatlib_mscp/Templates/MSCP SC9503-SPST-TTL Read Template ==
  Bus Creator : BusCreator  Inputs=8  OutDataTypeStr=Bus: MscpBus_SC9503_SPST_TTL
      settings: InheritFromInputs=off
  S-Function1 : S-Function  FunctionName=sg_mscp_SC9503_SPST_TTL_read  SFunctionDeploymentMode=off  EnableBusSupport=off
  exp0bank0 : slrealtimeethercatlib/EtherCAT PDO Receive  Priority=2  sig_name=Uninitialized Block  sig_offset=144  sig_type=uint8  type_size=8  sig_dim=1  device_id=0  sample_time=0.010000
  Out1 : Outport
  wires:
  S-Function1/8 -> Bus Creator/8  "Channel_08"
  S-Function1/7 -> Bus Creator/7  "Channel_07"
  S-Function1/6 -> Bus Creator/6  "Channel_06"
  S-Function1/5 -> Bus Creator/5  "Channel_05"
  S-Function1/4 -> Bus Creator/4  "Channel_04"
  S-Function1/3 -> Bus Creator/3  "Channel_03"
  S-Function1/2 -> Bus Creator/2  "Channel_02"
  S-Function1/1 -> Bus Creator/1  "Channel_01"
  Bus Creator/1 -> Out1/1
  exp0bank0/1 -> S-Function1/1

== system speedgoatlib_mscp/Templates/MSCP SC9503-SPST-TTL Write Template ==
  In2 : Inport  OutDataTypeStr=Bus: MscpBus_SC9503_SPST_TTL
  Bus Selector1 : BusSelector  OutputSignals=Channel_01,Channel_02,Channel_03,Channel_04,Channel_05,Channel_06,Channel_07,Channel_08
  S-Function1 : S-Function  FunctionName=sg_mscp_SC9503_SPST_TTL_write  SFunctionDeploymentMode=off  EnableBusSupport=off
  exp0bank0 : slrealtimeethercatlib/EtherCAT PDO Transmit  Priority=3  sig_name=Uninitialized Block  sig_offset=128  sig_type=uint8  type_size=8  sig_dim=1  device_id=0  sample_time=0.010000
  wires:
  S-Function1/1 -> exp0bank0/1
  Bus Selector1/8 -> S-Function1/8  "<Channel_08>"
  Bus Selector1/7 -> S-Function1/7  "<Channel_07>"
  Bus Selector1/6 -> S-Function1/6  "<Channel_06>"
  Bus Selector1/5 -> S-Function1/5  "<Channel_05>"
  Bus Selector1/4 -> S-Function1/4  "<Channel_04>"
  Bus Selector1/3 -> S-Function1/3  "<Channel_03>"
  Bus Selector1/2 -> S-Function1/2  "<Channel_02>"
  In2/1 -> Bus Selector1/1
  Bus Selector1/1 -> S-Function1/1  "<Channel_01>"

== system speedgoatlib_mscp/Templates/MSCP SC9601 Read Template ==
  Bus Creator : BusCreator  Inputs=14  OutDataTypeStr=Bus: MscpBus_SC9601
      settings: InheritFromInputs=off
  exp0bank{0..4} (5 alike) : slrealtimeethercatlib/EtherCAT PDO Receive  Priority=2  sig_name=Uninitialized Block  sig_offset=144  sig_type=uint8  type_size=8  sig_dim=1  device_id=0  sample_time=0.010000
  exp1bank{0..4} (5 alike) : slrealtimeethercatlib/EtherCAT PDO Receive  Priority=2  sig_name=Uninitialized Block  sig_offset=144  sig_type=uint8  type_size=8  sig_dim=1  device_id=0  sample_time=0.010000
  exp2bank{0..3} (4 alike) : slrealtimeethercatlib/EtherCAT PDO Receive  Priority=2  sig_name=Uninitialized Block  sig_offset=144  sig_type=uint8  type_size=8  sig_dim=1  device_id=0  sample_time=0.010000
  Out1 : Outport
  wires:
  exp2bank1/1 -> Bus Creator/12  "Channel_12"
  exp2bank0/1 -> Bus Creator/11  "Channel_11"
  exp1bank4/1 -> Bus Creator/10  "Channel_10"
  exp1bank3/1 -> Bus Creator/9  "Channel_09"
  exp1bank2/1 -> Bus Creator/8  "Channel_08"
  exp1bank1/1 -> Bus Creator/7  "Channel_07"
  exp1bank0/1 -> Bus Creator/6  "Channel_06"
  exp0bank4/1 -> Bus Creator/5  "Channel_05"
  exp0bank3/1 -> Bus Creator/4  "Channel_04"
  exp0bank2/1 -> Bus Creator/3  "Channel_03"
  exp0bank1/1 -> Bus Creator/2  "Channel_02"
  exp0bank0/1 -> Bus Creator/1  "Channel_01"
  Bus Creator/1 -> Out1/1
  exp2bank3/1 -> Bus Creator/14  "Fault_Insertion"
  exp2bank2/1 -> Bus Creator/13  "Termination"

== system speedgoatlib_mscp/Templates/MSCP SC9601 Write Template ==
  In1 : Inport  OutDataTypeStr=Bus: MscpBus_SC9601
  Bus Selector : BusSelector  OutputSignals=Channel_01,Channel_02,Channel_03,Channel_04,Channel_05,Channel_06,Channel_07,Channel_08,Channel_09,Channel_10,Channel_11,Channel_12,Termination,Fault_Insertion
  exp0bank{0..4} (5 alike) : slrealtimeethercatlib/EtherCAT PDO Transmit  Priority=3  sig_name=Uninitialized Block  sig_offset=128  sig_type=uint8  type_size=8  sig_dim=1  device_id=0  sample_time=0.010000
  exp1bank{0..4} (5 alike) : slrealtimeethercatlib/EtherCAT PDO Transmit  Priority=3  sig_name=Uninitialized Block  sig_offset=128  sig_type=uint8  type_size=8  sig_dim=1  device_id=0  sample_time=0.010000
  exp2bank{0..3} (4 alike) : slrealtimeethercatlib/EtherCAT PDO Transmit  Priority=3  sig_name=Uninitialized Block  sig_offset=128  sig_type=uint8  type_size=8  sig_dim=1  device_id=0  sample_time=0.010000
  wires:
  In1/1 -> Bus Selector/1
  Bus Selector/1 -> exp0bank0/1  "<Channel_01>"
  Bus Selector/4 -> exp0bank3/1  "<Channel_04>"
  Bus Selector/5 -> exp0bank4/1  "<Channel_05>"
  Bus Selector/6 -> exp1bank0/1  "<Channel_06>"
  Bus Selector/7 -> exp1bank1/1  "<Channel_07>"
  Bus Selector/8 -> exp1bank2/1  "<Channel_08>"
  Bus Selector/9 -> exp1bank3/1  "<Channel_09>"
  Bus Selector/10 -> exp1bank4/1  "<Channel_10>"
  Bus Selector/11 -> exp2bank0/1  "<Channel_11>"
  Bus Selector/2 -> exp0bank1/1  "<Channel_02>"
  Bus Selector/3 -> exp0bank2/1  "<Channel_03>"
  Bus Selector/12 -> exp2bank1/1  "<Channel_12>"
  Bus Selector/13 -> exp2bank2/1  "<Termination>"
  Bus Selector/14 -> exp2bank3/1  "<Fault_Insertion>"

== system speedgoatlib_mscp/Templates/MSCP Set SubDevice State ==
  Compare To Constant : simulink/Logic and Bit Operations/Compare To Constant  relop=~=  const=8  OutDataTypeStr=boolean
  Constant : Constant  Value=8  OutDataTypeStr=int32
  Get SubDevice State : slrealtimeethercatlib/Get SubDevice State  device_id=0  sample_time=1  subdevice_addr=0  selected_subdevice=Term 1 (EK1100)  timeout=500  subdevice_found=0
  Set SubDevice State : slrealtimeethercatlib/Set SubDevice State  device_id=0  sample_time=1  subdevice_addr=0  selected_subdevice=Term 1 (EK1100)  subdevice_found=0
  Terminator : Terminator
  Terminator1 : Terminator
  wires:
  Get SubDevice State/1 -> Compare To Constant/1
  Compare To Constant/1 -> Set SubDevice State/2
  Constant/1 -> Set SubDevice State/1
  Set SubDevice State/1 -> Terminator/1
  Set SubDevice State/2 -> Terminator1/1

== system speedgoatlib_mscp/Templates/MSCP SC2191 Read Advanced Template/Channel_01 ==
  Bus Creator : BusCreator  Inputs=6  OutDataTypeStr=Bus: MscpBus_SC2191_Channel_Advanced_Read
      settings: InheritFromInputs=off
  Vhigh : slrealtimeethercatlib/EtherCAT PDO Receive  Priority=2  sig_name=Uninitialized Block  sig_offset=144  sig_type=uint8  type_size=8  sig_dim=1  device_id=0  sample_time=0.010000
  Vhigh_Gain : slrealtimeethercatlib/EtherCAT PDO Receive  Priority=2  sig_name=Uninitialized Block  sig_offset=144  sig_type=uint8  type_size=8  sig_dim=1  device_id=0  sample_time=0.010000
  Vhigh_Offset : slrealtimeethercatlib/EtherCAT PDO Receive  Priority=2  sig_name=Uninitialized Block  sig_offset=144  sig_type=uint8  type_size=8  sig_dim=1  device_id=0  sample_time=0.010000
  Vlow : slrealtimeethercatlib/EtherCAT PDO Receive  Priority=2  sig_name=Uninitialized Block  sig_offset=144  sig_type=uint8  type_size=8  sig_dim=1  device_id=0  sample_time=0.010000
  Vlow_Gain : slrealtimeethercatlib/EtherCAT PDO Receive  Priority=2  sig_name=Uninitialized Block  sig_offset=144  sig_type=uint8  type_size=8  sig_dim=1  device_id=0  sample_time=0.010000
  Vlow_Offset : slrealtimeethercatlib/EtherCAT PDO Receive  Priority=2  sig_name=Uninitialized Block  sig_offset=144  sig_type=uint8  type_size=8  sig_dim=1  device_id=0  sample_time=0.010000
  Out1 : Outport
  wires:
  Vhigh/1 -> Bus Creator/2
  Vlow/1 -> Bus Creator/1
  Bus Creator/1 -> Out1/1
  Vlow_Offset/1 -> Bus Creator/3
  Vlow_Gain/1 -> Bus Creator/4
  Vhigh_Offset/1 -> Bus Creator/5
  Vhigh_Gain/1 -> Bus Creator/6

== system speedgoatlib_mscp/Templates/MSCP SC2191 Read Advanced Template/Channel_02 ==
  Bus Creator : BusCreator  Inputs=6  OutDataTypeStr=Bus: MscpBus_SC2191_Channel_Advanced_Read
      settings: InheritFromInputs=off
  Vhigh : slrealtimeethercatlib/EtherCAT PDO Receive  Priority=2  sig_name=Uninitialized Block  sig_offset=144  sig_type=uint8  type_size=8  sig_dim=1  device_id=0  sample_time=0.010000
  Vhigh_Gain : slrealtimeethercatlib/EtherCAT PDO Receive  Priority=2  sig_name=Uninitialized Block  sig_offset=144  sig_type=uint8  type_size=8  sig_dim=1  device_id=0  sample_time=0.010000
  Vhigh_Offset : slrealtimeethercatlib/EtherCAT PDO Receive  Priority=2  sig_name=Uninitialized Block  sig_offset=144  sig_type=uint8  type_size=8  sig_dim=1  device_id=0  sample_time=0.010000
  Vlow : slrealtimeethercatlib/EtherCAT PDO Receive  Priority=2  sig_name=Uninitialized Block  sig_offset=144  sig_type=uint8  type_size=8  sig_dim=1  device_id=0  sample_time=0.010000
  Vlow_Gain : slrealtimeethercatlib/EtherCAT PDO Receive  Priority=2  sig_name=Uninitialized Block  sig_offset=144  sig_type=uint8  type_size=8  sig_dim=1  device_id=0  sample_time=0.010000
  Vlow_Offset : slrealtimeethercatlib/EtherCAT PDO Receive  Priority=2  sig_name=Uninitialized Block  sig_offset=144  sig_type=uint8  type_size=8  sig_dim=1  device_id=0  sample_time=0.010000
  Out1 : Outport
  wires:
  Vhigh_Gain/1 -> Bus Creator/6
  Vhigh_Offset/1 -> Bus Creator/5
  Vlow_Gain/1 -> Bus Creator/4
  Vlow_Offset/1 -> Bus Creator/3
  Bus Creator/1 -> Out1/1
  Vlow/1 -> Bus Creator/1
  Vhigh/1 -> Bus Creator/2

== system speedgoatlib_mscp/Templates/MSCP SC2191 Read Advanced Template/Channel_03 ==
  Bus Creator : BusCreator  Inputs=6  OutDataTypeStr=Bus: MscpBus_SC2191_Channel_Advanced_Read
      settings: InheritFromInputs=off
  Vhigh : slrealtimeethercatlib/EtherCAT PDO Receive  Priority=2  sig_name=Uninitialized Block  sig_offset=144  sig_type=uint8  type_size=8  sig_dim=1  device_id=0  sample_time=0.010000
  Vhigh_Gain : slrealtimeethercatlib/EtherCAT PDO Receive  Priority=2  sig_name=Uninitialized Block  sig_offset=144  sig_type=uint8  type_size=8  sig_dim=1  device_id=0  sample_time=0.010000
  Vhigh_Offset : slrealtimeethercatlib/EtherCAT PDO Receive  Priority=2  sig_name=Uninitialized Block  sig_offset=144  sig_type=uint8  type_size=8  sig_dim=1  device_id=0  sample_time=0.010000
  Vlow : slrealtimeethercatlib/EtherCAT PDO Receive  Priority=2  sig_name=Uninitialized Block  sig_offset=144  sig_type=uint8  type_size=8  sig_dim=1  device_id=0  sample_time=0.010000
  Vlow_Gain : slrealtimeethercatlib/EtherCAT PDO Receive  Priority=2  sig_name=Uninitialized Block  sig_offset=144  sig_type=uint8  type_size=8  sig_dim=1  device_id=0  sample_time=0.010000
  Vlow_Offset : slrealtimeethercatlib/EtherCAT PDO Receive  Priority=2  sig_name=Uninitialized Block  sig_offset=144  sig_type=uint8  type_size=8  sig_dim=1  device_id=0  sample_time=0.010000
  Out1 : Outport
  wires:
  Vhigh/1 -> Bus Creator/2
  Vlow/1 -> Bus Creator/1
  Bus Creator/1 -> Out1/1
  Vlow_Offset/1 -> Bus Creator/3
  Vlow_Gain/1 -> Bus Creator/4
  Vhigh_Offset/1 -> Bus Creator/5
  Vhigh_Gain/1 -> Bus Creator/6

== system speedgoatlib_mscp/Templates/MSCP SC2191 Read Advanced Template/Channel_04 ==
  Bus Creator : BusCreator  Inputs=6  OutDataTypeStr=Bus: MscpBus_SC2191_Channel_Advanced_Read
      settings: InheritFromInputs=off
  Vhigh : slrealtimeethercatlib/EtherCAT PDO Receive  Priority=2  sig_name=Uninitialized Block  sig_offset=144  sig_type=uint8  type_size=8  sig_dim=1  device_id=0  sample_time=0.010000
  Vhigh_Gain : slrealtimeethercatlib/EtherCAT PDO Receive  Priority=2  sig_name=Uninitialized Block  sig_offset=144  sig_type=uint8  type_size=8  sig_dim=1  device_id=0  sample_time=0.010000
  Vhigh_Offset : slrealtimeethercatlib/EtherCAT PDO Receive  Priority=2  sig_name=Uninitialized Block  sig_offset=144  sig_type=uint8  type_size=8  sig_dim=1  device_id=0  sample_time=0.010000
  Vlow : slrealtimeethercatlib/EtherCAT PDO Receive  Priority=2  sig_name=Uninitialized Block  sig_offset=144  sig_type=uint8  type_size=8  sig_dim=1  device_id=0  sample_time=0.010000
  Vlow_Gain : slrealtimeethercatlib/EtherCAT PDO Receive  Priority=2  sig_name=Uninitialized Block  sig_offset=144  sig_type=uint8  type_size=8  sig_dim=1  device_id=0  sample_time=0.010000
  Vlow_Offset : slrealtimeethercatlib/EtherCAT PDO Receive  Priority=2  sig_name=Uninitialized Block  sig_offset=144  sig_type=uint8  type_size=8  sig_dim=1  device_id=0  sample_time=0.010000
  Out1 : Outport
  wires:
  Vhigh_Gain/1 -> Bus Creator/6
  Vhigh_Offset/1 -> Bus Creator/5
  Vlow_Gain/1 -> Bus Creator/4
  Vlow_Offset/1 -> Bus Creator/3
  Bus Creator/1 -> Out1/1
  Vlow/1 -> Bus Creator/1
  Vhigh/1 -> Bus Creator/2

== system speedgoatlib_mscp/Templates/MSCP SC2191 Read Advanced Template/Channel_05 ==
  Bus Creator : BusCreator  Inputs=6  OutDataTypeStr=Bus: MscpBus_SC2191_Channel_Advanced_Read
      settings: InheritFromInputs=off
  Vhigh : slrealtimeethercatlib/EtherCAT PDO Receive  Priority=2  sig_name=Uninitialized Block  sig_offset=144  sig_type=uint8  type_size=8  sig_dim=1  device_id=0  sample_time=0.010000
  Vhigh_Gain : slrealtimeethercatlib/EtherCAT PDO Receive  Priority=2  sig_name=Uninitialized Block  sig_offset=144  sig_type=uint8  type_size=8  sig_dim=1  device_id=0  sample_time=0.010000
  Vhigh_Offset : slrealtimeethercatlib/EtherCAT PDO Receive  Priority=2  sig_name=Uninitialized Block  sig_offset=144  sig_type=uint8  type_size=8  sig_dim=1  device_id=0  sample_time=0.010000
  Vlow : slrealtimeethercatlib/EtherCAT PDO Receive  Priority=2  sig_name=Uninitialized Block  sig_offset=144  sig_type=uint8  type_size=8  sig_dim=1  device_id=0  sample_time=0.010000
  Vlow_Gain : slrealtimeethercatlib/EtherCAT PDO Receive  Priority=2  sig_name=Uninitialized Block  sig_offset=144  sig_type=uint8  type_size=8  sig_dim=1  device_id=0  sample_time=0.010000
  Vlow_Offset : slrealtimeethercatlib/EtherCAT PDO Receive  Priority=2  sig_name=Uninitialized Block  sig_offset=144  sig_type=uint8  type_size=8  sig_dim=1  device_id=0  sample_time=0.010000
  Out1 : Outport
  wires:
  Vhigh/1 -> Bus Creator/2
  Vlow/1 -> Bus Creator/1
  Bus Creator/1 -> Out1/1
  Vlow_Offset/1 -> Bus Creator/3
  Vlow_Gain/1 -> Bus Creator/4
  Vhigh_Offset/1 -> Bus Creator/5
  Vhigh_Gain/1 -> Bus Creator/6

== system speedgoatlib_mscp/Templates/MSCP SC2191 Read Advanced Template/Channel_06 ==
  Bus Creator : BusCreator  Inputs=6  OutDataTypeStr=Bus: MscpBus_SC2191_Channel_Advanced_Read
      settings: InheritFromInputs=off
  Vhigh : slrealtimeethercatlib/EtherCAT PDO Receive  Priority=2  sig_name=Uninitialized Block  sig_offset=144  sig_type=uint8  type_size=8  sig_dim=1  device_id=0  sample_time=0.010000
  Vhigh_Gain : slrealtimeethercatlib/EtherCAT PDO Receive  Priority=2  sig_name=Uninitialized Block  sig_offset=144  sig_type=uint8  type_size=8  sig_dim=1  device_id=0  sample_time=0.010000
  Vhigh_Offset : slrealtimeethercatlib/EtherCAT PDO Receive  Priority=2  sig_name=Uninitialized Block  sig_offset=144  sig_type=uint8  type_size=8  sig_dim=1  device_id=0  sample_time=0.010000
  Vlow : slrealtimeethercatlib/EtherCAT PDO Receive  Priority=2  sig_name=Uninitialized Block  sig_offset=144  sig_type=uint8  type_size=8  sig_dim=1  device_id=0  sample_time=0.010000
  Vlow_Gain : slrealtimeethercatlib/EtherCAT PDO Receive  Priority=2  sig_name=Uninitialized Block  sig_offset=144  sig_type=uint8  type_size=8  sig_dim=1  device_id=0  sample_time=0.010000
  Vlow_Offset : slrealtimeethercatlib/EtherCAT PDO Receive  Priority=2  sig_name=Uninitialized Block  sig_offset=144  sig_type=uint8  type_size=8  sig_dim=1  device_id=0  sample_time=0.010000
  Out1 : Outport
  wires:
  Vhigh_Gain/1 -> Bus Creator/6
  Vhigh_Offset/1 -> Bus Creator/5
  Vlow_Gain/1 -> Bus Creator/4
  Vlow_Offset/1 -> Bus Creator/3
  Bus Creator/1 -> Out1/1
  Vlow/1 -> Bus Creator/1
  Vhigh/1 -> Bus Creator/2
